simulink model "pend_on_cart"  (R2021a)
settings: Solver=VariableStepAuto  StartTime=0.0  StopTime=1  RelTol=1e-3
(part 3 of 3)

== matlab function pend_on_cart/MATLAB Function ==
  data: x input; dx output; theta input; alpha input; dx input; dtheta input; dalpha input; u0 input; u1 input; dtheta output; dalpha output; ddx output; ddtheta output; ddalpha output
function [dx, dtheta, dalpha, ddx, ddtheta, ddalpha] = pend_on_cart(x, theta, alpha, dx, dtheta, dalpha,u0, u1)

B = [(353160*sin(theta + 2*alpha) - 1059480*sin(2*theta + alpha) + 18000*cos(2*theta + 2*alpha) + 794610*sin(theta) - 1118340*sin(alpha) - 42125)/(353160*sin(theta + 2*alpha) - 1059480*sin(2*theta + alpha) + 18000*cos(2*theta + 2*alpha) + 1059480*sin(theta) - 1153656*sin(alpha) + (135*972361^(1/2)*cos(atan(981/100) + 2*theta))/2 + 3*972361^(1/2)*cos(atan(981/100) - 2*alpha) - 49550), (353160*sin(theta + 2*alpha) - 4237920*sin(theta - alpha) + 18000*cos(2*theta + 2*alpha) + 794610*sin(theta) - 4237920*sin(theta + alpha) + 12713760*sin(2*theta) - 1080*1002361^(1/2)*cos(2*theta - atan(981/200) + alpha) + 1140*1002361^(1/2)*cos(atan(981/200) + alpha) - 42125)/(706320*sin(theta + 2*alpha) - 2118960*sin(2*theta + alpha) + 36000*cos(2*theta + 2*alpha) + 2118960*sin(theta) - 2307312*sin(alpha) + 135*972361^(1/2)*cos(atan(981/100) + 2*theta) + 6*972361^(1/2)*cos(atan(981/100) - 2*alpha) - 99100);
                           (2*(4237920*sin(theta + alpha) - 360*972361^(1/2)*cos(theta - atan(981/100) + 2*alpha) + 810*972361^(1/2)*cos(atan(981/100) + theta)))/(706320*sin(theta + 2*alpha) - 2118960*sin(2*theta + alpha) + 36000*cos(2*theta + 2*alpha) + 2118960*sin(theta) - 2307312*sin(alpha) + 135*972361^(1/2)*cos(atan(981/100) + 2*theta) + 6*972361^(1/2)*cos(atan(981/100) - 2*alpha) - 99100),                                                                              (2*(2025*1134410161^(1/2)*cos(atan(33681/20) + theta) - 2160*972361^(1/2)*cos(atan(981/100) + theta - alpha) + 1440*9083749^(1/2)*cos(theta - atan(2943/650) + alpha) - 180*972361^(1/2)*cos(theta - atan(981/100) + 2*alpha)))/(706320*sin(theta + 2*alpha) - 2118960*sin(2*theta + alpha) + 36000*cos(2*theta + 2*alpha) + 2118960*sin(theta) - 2307312*sin(alpha) + 135*972361^(1/2)*cos(atan(981/100) + 2*theta) + 6*972361^(1/2)*cos(atan(981/100) - 2*alpha) - 99100);
                        -(2*(4237920*sin(theta + alpha) + 1080*972361^(1/2)*cos(atan(981/100) + 2*theta + alpha) - 1140*972361^(1/2)*cos(atan(981/100) - alpha)))/(706320*sin(theta + 2*alpha) - 2118960*sin(2*theta + alpha) + 36000*cos(2*theta + 2*alpha) + 2118960*sin(theta) - 2307312*sin(alpha) + 135*972361^(1/2)*cos(atan(981/100) + 2*theta) + 6*972361^(1/2)*cos(atan(981/100) - 2*alpha) - 99100),                                                                                      (2*(67806720*sin(theta) - 2118960*sin(theta + alpha) - 540*972361^(1/2)*cos(atan(981/100) + 2*theta + alpha) + 6480*972361^(1/2)*cos(atan(981/100) + 2*theta) + 570*972361^(1/2)*cos(atan(981/100) - alpha) - 2904000))/(706320*sin(theta + 2*alpha) - 2118960*sin(2*theta + alpha) + 36000*cos(2*theta + 2*alpha) + 2118960*sin(theta) - 2307312*sin(alpha) + 135*972361^(1/2)*cos(atan(981/100) + 2*theta) + 6*972361^(1/2)*cos(atan(981/100) - 2*alpha) - 99100)];
%dx = dx;
%dtheta = dtheta;
%dalpha = dalpha;
ddx = (132435*sin(2*theta) - 5886*sin(2*alpha) + 300*sin(theta + 2*alpha)*dtheta^2 + 2250*sin(2*theta + alpha)*dalpha^2 - 14175*sin(theta)*dtheta^2 - 2575*sin(alpha)*dalpha^2)/(100*(360*cos(2*theta + 2*alpha) + 135*cos(2*theta) + 6*cos(2*alpha) - 991))+ B(1,:)*[u0;u1];
ddtheta = -(35316*sin(theta + 2*alpha) + 105948*sin(theta) + 2175*sin(theta + alpha)*dalpha^2 - 675*sin(2*theta)*dtheta^2 + 225*sin(theta - alpha)*dalpha^2 - 1800*sin(2*theta + 2*alpha)*dtheta^2)/(1800*cos(2*theta + 2*alpha) + 675*cos(2*theta) + 30*cos(2*alpha) - 4955)+ B(2,:)*[u0;u1];
ddalpha = (529740*sin(2*theta + alpha) + 576828*sin(alpha) - 55950*sin(theta + alpha)*dtheta^2 + 150*sin(2*alpha)*dalpha^2 + 450*sin(theta - alpha)*dtheta^2 + 9000*sin(2*theta + 2*alpha)*dalpha^2)/(25*(360*cos(2*theta + 2*alpha) + 135*cos(2*theta) + 6*cos(2*alpha) - 991))+ B(3,:)*[u0;u1];
